simulink model "DAB_Tri_Trap"  (R2022b)
settings: Solver=ode23t  StartTime=0.0  StopTime=1/fsw*10000  MaxStep=1/100000  RelTol=1e-7  AbsTol=1e-7
StartFcn:
  | tic
StopFcn:
  | toc
undefined symbols (not defined in the file): DiscIntNeverNeededParam, fsw, L, n, ntemp, period, R_Load, tau, ts_pwm, Vdc1, Vth
libraries: nesl_utility x15, fl_lib x12, ee_lib x8, simulink x5, slpidlib x1
(part 2 of 2)

== stateflow chart DAB_Tri_Trap/DAB_Trap_Tri_Controller/PWM_Peripheral/PWM Feedback Controller/Subsystem/Commutation Logic ==
  state A
    entry:
    test = 0;
    mt = 0;
    mb = 0;
  state B
    entry:
    test = 1;
    mt = 1;
    mb = 0;
  state C
    entry:
    test = 2;
    mt = 1;
    mb = 1;
  state D
    entry:
    test = 3;
    mt = 2;
    mb = 1;
  state H
    entry:
    test = 7;
    mt = 0;
    mb = 3;
  state G
    entry:
    test = 6;
    mt = 3;
    mb = 3;
  state F
    entry:
    test = 5;
    mt = 3;
    mb = 2;
  state E
    entry:
    test = 4;
    mt = 2;
    mb = 2;
  (default) -> A
  B -> C : [mode_bot == 1]
  A -> B : [mode_top == 1 && ...
      | mode_bot == 0]
  C -> D : [mode_top == 2]
  H -> A : [I_L >= 0]
  D -> E : [I_L <= 0]
  G -> H : [mode_top == 0]
  F -> G : [mode_bot == 3]
  E -> F : [mode_top == 3]
  data: mode_top input; mode_bot input; test output int8; I_L input; mt output int8; mb output int8

== matlab function DAB_Tri_Trap/DAB_Trap_Tri_Controller/CPU_Based_Control/Omega_tri ==
  data: omega1 output; V1 input; V2 input; delta input; omega2 output
function [omega1, omega2] = fcn(V1,V2,delta)

if V1 < V2
    omega1 = pi/2-(abs(delta)*V2)/(V2-V1);
    omega2 = abs(delta)+omega1;
else
    omega2 = pi/2+(abs(delta)*V1)/(V2-V1);
    omega1 = abs(delta)+omega2;
end

== matlab function DAB_Tri_Trap/DAB_Trap_Tri_Controller/CPU_Based_Control/delta_estimate ==
  data: I input; V1 input; V2 input; ex1 input; ex2 input; ex3 input; fsw input; tau_blank input; L input; delta_est output; trap_mode input; delta_max input
function delta_est = fcn(I,V1,V2,ex1,ex2,ex3,fsw,tau_blank,L, trap_mode, delta_max)

if trap_mode

    if (ex3*(4*fsw^2*tau_blank^2+1) - 4*fsw*(abs(I)*L*ex2+tau_blank*ex3)) <= 0
        delta_est = delta_max;
    else
        delta_est = sign(I)*pi*(ex1*(1-2*tau_blank*fsw)/(2*ex2) - (V1+V2)*sqrt(ex3*(4*fsw^2*tau_blank^2+1) - 4*fsw*(abs(I)*L*ex2+tau_blank*ex3))/(2*sqrt(V1)*ex2));
    end

else

    if V1 < V2
        delta_est = sign(I)*pi*sqrt(abs(I)*L*fsw*(V2-V1))/V1;
    else
        delta_est = sign(I)*pi*sqrt(abs(I)*L*fsw*(V1-V2))/sqrt(V1*V2);
    end

end

== matlab function DAB_Tri_Trap/DAB_Trap_Tri_Controller/CPU_Based_Control/Omega_trap ==
  data: tau input; omega1 output; fsw input; V1 input; V2 input; delta input; omega2 output
function [omega1, omega2] = fcn(tau,fsw,V1,V2,delta)

if V1 <= V2
    omega1 = (pi*(V1-V2)+2*V2*(abs(delta)+2*pi*tau*fsw))/(2*(V1+V2));
    omega2 = abs(delta)-omega1+2*pi*tau*fsw;
else
    omega2 = (pi*(V2-V1)+2*V1*(abs(delta)+2*pi*tau*fsw))/(2*(V1+V2));
    omega1 = abs(delta)-omega2+2*pi*tau*fsw;
end

== stateflow chart DAB_Tri_Trap/DAB_Trap_Tri_Controller/PWM_Peripheral/PWM Feedback Controller/Switch Case Action Subsystem/Commutation Logic for V1 > V1 ==
  state A
    entry:
    test = 0;
    mt = 0;
    mb = 0;
  state B
    entry:
    test = 1;
    mt = 1;
    mb = 1;
  state C
    entry:
    test = 2;
    mt = 2;
  state F
    entry:
    test = 5;
    mt = 0;
  state E
    entry:
    test = 4;
    mt = 3;
    mb = 3;
  state D
    entry:
    test = 3;
    mb = 2;
  (default) -> A
  B -> C : [mode_top == 2]
  A -> B : [mode_top == 1 && ...
      | mode_bot ==1]
  F -> A : [I_L >= 0]
  C -> D : [I_L <= 0]
  E -> F : [mode_top == 0]
  D -> E : [mode_top == 3 && ...
      | mode_bot == 3]
  data: mode_top input; mode_bot input; test output int8; I_L input; mt output int8; mb output int8
